simulink model "untitled4"  (R2015a)
settings: Solver=ode45  StartTime=0.0  StopTime=10.0  RelTol=1e-3
libraries: commchan3 x1, dsparch4 x1, commsink2 x1, commutil2 x1, dspsigops x1, commrandsrc2 x1
settings Model: Creator=TaD  LastModifiedBy=TaD

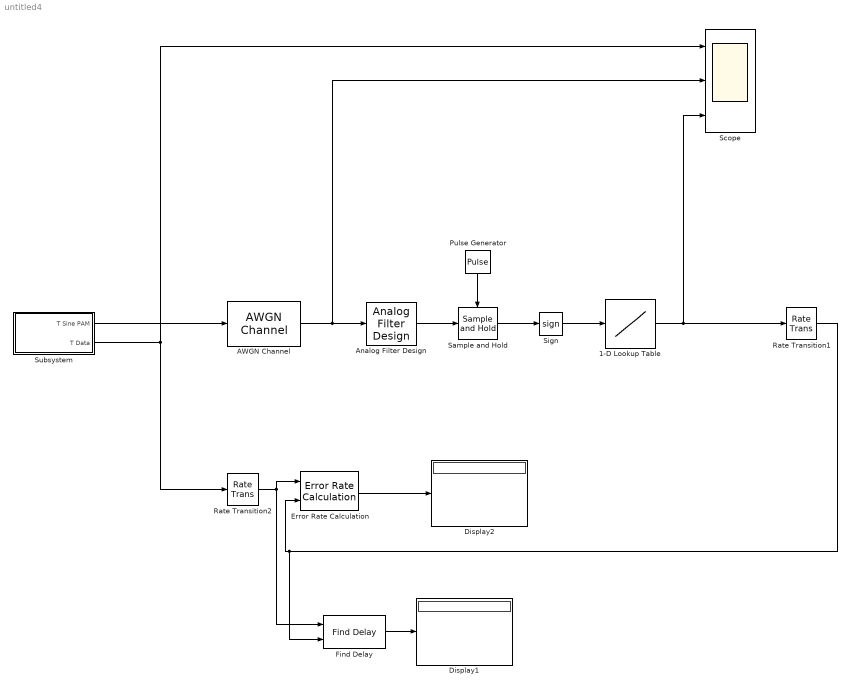
== system untitled4 ==
  1-D Lookup Table : Lookup_n-D  NumberOfTableDimensions=1  BreakpointsForDimension1=[-49:50]  Table=[zeros(1,50) 1:50]  InternalRulePriority=Speed  RndMeth=Simplest  InputSameDT=on
  AWGN Channel : commchan3/AWGN Channel  InputProcessing=Columns as channels (frame based)  seed=67  noiseMode=Variance from mask  EbNodB=10  EsNodB=10  SNRdB=10  bitsPerSym=1  Ps=1  Tsym=1  variance=0.5
  Analog Filter Design : dsparch4/Analog Filter Design  method=Chebyshev I  filttype=Lowpass  N=9  Wlo=600  Whi=80  Rp=0.1  Rs=40
  Display1 : Display
  Display2 : Display
  Error Rate Calculation : commsink2/Error Rate Calculation  N=0  st_delay=0  cp_mode=Entire frame  subframe=[]  PMode=Port  WsName=ErrorVec  RsMode2=off  stop=off  numErr=100  maxBits=1e6
  Find Delay : commutil2/Find Delay  corrLength=200  chgSigOP=off  stopUpdate=off  numConstDelay=3
  Pulse Generator : DiscretePulseGenerator  Amplitude=5  Period=10  PulseWidth=5  SampleTime=2e-6
  Rate Transition1 : RateTransition  Deterministic=off  OutPortSampleTime=1/2000
  Rate Transition2 : RateTransition  Deterministic=off  OutPortSampleTime=1/2000
  Sample and Hold : dspsigops/Sample and Hold  trig=Rising edge  initCond=0  latchinput=off
  Scope : Scope  NumInputPorts=3
      settings: YMin=-5~-5~-5  YMax=5~5~5
  Sign : Signum
  Subsystem : Subsystem
  wires:
  Rate Transition2/1 -> Find Delay/1, Error Rate Calculation/1
  Sample and Hold/1 -> Sign/1
  Sign/1 -> 1-D Lookup Table/1
  1-D Lookup Table/1 -> Rate Transition1/1, Scope/3
  Pulse Generator/1 -> Sample and Hold/Trigger
  Rate Transition1/1 -> Find Delay/2, Error Rate Calculation/2
  Find Delay/1 -> Display1/1
  Error Rate Calculation/1 -> Display2/1
  AWGN Channel/1 -> Analog Filter Design/1, Scope/2
  Analog Filter Design/1 -> Sample and Hold/1
  Subsystem/1("T Sine PAM ") -> AWGN Channel/1
  Subsystem/2(T Data) -> Rate Transition2/1, Scope/1

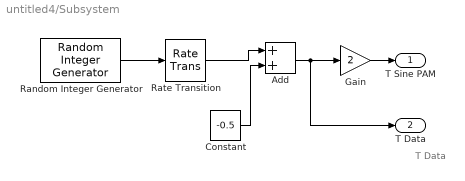
== system untitled4/Subsystem ==
  note: T Data
  Add : Sum
  Constant : Constant  Value=-0.5  SampleTime=1/1000
  Gain : Gain  Gain=2
  Random Integer Generator : commrandsrc2/Random Integer Generator  mul=2  seed=37  Ts=2e-4  frameBased=off  sampPerFrame=1  orient=off  outDataType=double
  Rate Transition : RateTransition  Deterministic=off  OutPortSampleTimeOpt=Multiple of input port sample time  OutPortSampleTime=1
  "T Sine PAM " : Outport
  T Data : Outport  Port=2
  wires:
  Rate Transition/1 -> Add/1
  Random Integer Generator/1 -> Rate Transition/1
  Add/1 -> T Data/1, Gain/1
  Constant/1 -> Add/2
  Gain/1 -> "T Sine PAM "/1
